simulink model "big2"  (R2023b)
settings: Solver=VariableStepAuto  StartTime=0.0  StopTime=500  RelTol=1e-3
libraries: simulink x2, aerolibasang x2, simulink_extras x2, aerolibanim x1
(part 2 of 3)

== matlab function big2/Subsystem1/Subsystem/MATLAB Function4 ==
  data: F input; V_dot output; g input; m input; theta input; psi input; P input; R input; U input; W input
function V_dot = fcn(F,g,m,theta,psi,P,R,U,W)
    if m == 0
        V_dot = NaN;
        warning('Mass (m) is zero, returning NaN.');
        return;
    end
    % Ensure theta and psi are valid
    if isnan(theta) || isnan(psi)
        V_dot = NaN;
        warning('Theta or Psi is NaN, returning NaN.');
        return;
    end
    V_dot = P*W - R*U + g*cos(theta)*sin(psi) + F/m;
    % V_dot = 0;

== matlab function big2/Subsystem1/Subsystem/MATLAB Function5 ==
  data: F input; W_dot output; g input; m input; theta input; psi input; P input; Q input; U input; V input
function W_dot = fcn(F,g,m,theta,psi,P,Q,U,V)
W_dot = Q*U - P*V + g*cos(theta)*cos(psi) + F/m;

== matlab function big2/Subsystem1/Subsystem/MATLAB Function6 ==
  data: phi input; euler_rates output; theta input; P input; Q input; R input
function euler_rates = fcn(phi, theta, P, Q, R)
if abs(cos(theta)) < 1e-6
    error('Theta is near ±pi/2, causing a singularity.');
end

T = [1, sin(phi)*tan(theta), cos(phi)*tan(theta);
     0, cos(phi), -sin(phi);
     0, sin(phi)/cos(theta), cos(phi)/cos(theta)];

angular_velocity = [P; Q; R];

euler_rates = T * angular_velocity;
end

== matlab function big2/Subsystem/Subsystem1/MATLAB Function ==
  data: alpha input; c_x output; el input
function c_x = compute_cx_fixed(alpha, el)
    data = [
    -0.099, -0.081, -0.081, -0.063, -0.025, 0.044, 0.097, 0.113, 0.145, 0.167, 0.174, 0.166;
    -0.048, -0.038, -0.040, -0.021, 0.016, 0.083, 0.127, 0.137, 0.162, 0.177, 0.179, 0.167;
    -0.022, -0.020, -0.021, -0.004, 0.032, 0.094, 0.128, 0.130, 0.154, 0.161, 0.155, 0.138;
    -0.040, -0.038, -0.039, -0.025, 0.006, 0.062, 0.087, 0.085, 0.100, 0.110, 0.104, 0.091;
    -0.083, -0.073, -0.076, -0.072, -0.046, 0.012, 0.024, 0.025, 0.043, 0.053, 0.047, 0.040
    ];
    % Scale Alpha and EL
    scaled_alpha = 0.2 * alpha;
    k = floor(scaled_alpha);
    k = max(-2, min(k, 8)); % Constrain within bounds
    da = scaled_alpha - k;
    l = k + sign(1.1 * da);
    l = max(-2, min(l, 8)); % Constrain within bounds

    % Adjust indices for 1-based indexing
    k_index = k + 3; % MATLAB 1-based (add 3 instead of 2 for [-2, 8])
    l_index = l + 3;

    % Scale EL
    scaled_el = el / 12.5;
    m = floor(scaled_el);
    m = max(-2, min(m, 2)); % Constrain within bounds
    de = scaled_el - m;
    n = m + sign(1.1 * de);
    n = max(-2, min(n, 2)); % Constrain within bounds

    % Adjust indices for 1-based indexing
    m_index = m + 3; % MATLAB 1-based (add 3 instead of 2 for [-2, 2])
    n_index = n + 3;

    % Ensure indices are within valid ranges
    assert(m_index >= 1 && m_index <= size(data, 1), 'm_index out of bounds');
    assert(n_index >= 1 && n_index <= size(data, 1), 'n_index out of bounds');
    assert(k_index >= 1 && k_index <= size(data, 2), 'k_index out of bounds');
    assert(l_index >= 1 && l_index <= size(data, 2), 'l_index out of bounds');

    % Interpolate values
    t = data(m_index, k_index); % Top-left
    u = data(n_index, k_index); % Bottom-left
    v = t + abs(da) * (data(m_index, l_index) - t); % Interpolation along top row
    w = u + abs(da) * (data(n_index, l_index) - u); % Interpolation along bottom row
    c_x = v + (w - v) * abs(de); % Final interpolation
end

== matlab function big2/Subsystem1/Subsystem/MATLAB Function7 ==
  data: U input; V input; W input; phi input; vel_dot output; theta input; psi input
function vel_dot = fcn(U, V, W, phi, theta, psi)
% This function computes [x_dot_e; y_dot_e; -h_dot] using the given equation.
% Inputs:
% U, V, W - Body frame velocities (m/s)
% phi     - Roll angle (rad)
% theta   - Pitch angle (rad)
% psi     - Yaw angle (rad)

% Rotation matrices
R_psi = [cos(psi), -sin(psi), 0;
         sin(psi),  cos(psi), 0;
         0,         0,        1];

R_theta = [cos(theta), 0, sin(theta);
           0,          1, 0;
          -sin(theta), 0, cos(theta)];

R_phi = [1, 0,       0;
         0, cos(phi), -sin(phi);
         0, sin(phi),  cos(phi)];

% Overall transformation matrix
R = R_psi * R_theta * R_phi;

% Body velocities vector
body_velocities = [U; V; W];

% Compute [x_dot_e; y_dot_e; -h_dot]
vel_dot = R * body_velocities;
end

== matlab function big2/Subsystem/Subsystem2/MATLAB Function ==
  data: alpha input; Cxq output
function Cxq = lookup_Cxq(alpha)
    % Initialize output
    Cxq = 0; % Ensure Cxq is scalar and fixed size

    % Declare persistent variables to hold constant data
    persistent alpha_values Cxq_values num_points

    if isempty(alpha_values)
        % Initialize the lookup table values as constants
        alpha_values = [-10, -5, 0, 5, 10, 15, 20, 25, 30, 35, 40, 45];
        Cxq_values  = [-0.267, -0.110, 0.308, 1.34, 2.08, 2.91, 2.76, 2.05, 1.50, 1.49, 1.83, 1.21];
        num_points = length(alpha_values);
    end

    % Handle values outside the table range
    if alpha <= alpha_values(1)
        Cxq = Cxq_values(1);
    elseif alpha >= alpha_values(num_points)
        Cxq = Cxq_values(num_points);
    else
        % Find the interval containing alpha
        idx = int32(1);
        for i = int32(1):(num_points - 1)
            if alpha_values(i) <= alpha && alpha < alpha_values(i+1)
                idx = i;
                break;
            end
        end

        % Get the two points for interpolation
        x1 = alpha_values(idx);
        x2 = alpha_values(idx + 1);
        y1 = Cxq_values(idx);
        y2 = Cxq_values(idx + 1);

        % Linear interpolation
        Cxq = y1 + ((y2 - y1) * (alpha - x1)) / (x2 - x1);
    end
end

== matlab function big2/Subsystem/Subsystem2/MATLAB Function1 ==
  data: alpha input; CYr output
function CYr = lookup_CYr(alpha)
    % Initialize output
    CYr = 0; % Ensure Cxq is scalar and fixed size

    % Declare persistent variables to hold constant data
    persistent alpha_values CYr_values num_points

    if isempty(alpha_values)
        % Initialize the lookup table values as constants
        alpha_values = [-Inf, -10, -5, 0, 5, 10, 15, 20, 25, 30, 35, 40, 45, Inf];
        CYr_values = [.882,.882, .852, .876, .958, .962, .974, .819, .483, .590, 1.21, -.493, -1.04, -1.04];
        num_points = length(alpha_values);
    end

    % Handle values outside the table range
    if alpha <= alpha_values(1)
        CYr = CYr_values(1);
    elseif alpha >= alpha_values(num_points)
        CYr = CYr_values(num_points);
    else
        % Find the interval containing alpha
        idx = int32(1);
        for i = int32(1):(num_points - 1)
            if alpha_values(i) <= alpha && alpha < alpha_values(i+1)
                idx = i;
                break;
            end
        end

        % Get the two points for interpolation
        x1 = alpha_values(idx);
        x2 = alpha_values(idx + 1);
        y1 = CYr_values(idx);
        y2 = CYr_values(idx + 1);

        % Linear interpolation
        CYr = y1 + ((y2 - y1) * (alpha - x1)) / (x2 - x1);
    end
end

== matlab function big2/Subsystem/Subsystem2/MATLAB Function2 ==
  data: alpha input; CYp output
function CYp = lookup_CYp(alpha)
    % Initialize output
    CYp = 0; % Ensure CYp is scalar and fixed size

    % Declare persistent variables to hold constant data
    persistent alpha_values CYp_values num_points

    if isempty(alpha_values)
        % Initialize the lookup table values as constants
        alpha_values = [-10, -5, 0, 5, 10, 15, 20, 25, 30, 35, 40, 45];
        CYp_values  = [-0.108, -0.188, 0.110, 0.258, 0.226, 0.344, 0.362, 0.611, 0.529, 0.298, -2.27, -2.27];
        num_points = length(alpha_values);
    end

    % Handle values outside the table range
    if alpha <= alpha_values(1)
        CYp = CYp_values(1);
    elseif alpha >= alpha_values(num_points)
        CYp = CYp_values(num_points);
    else
        % Find the interval containing alpha
        idx = int32(1);
        for i = int32(1):(num_points - 1)
            if alpha_values(i) <= alpha && alpha < alpha_values(i+1)
                idx = i;
                break;
            end
        end

        % Get the two points for interpolation
        x1 = alpha_values(idx);
        x2 = alpha_values(idx + 1);
        y1 = CYp_values(idx);
        y2 = CYp_values(idx + 1);

        % Linear interpolation
        CYp = y1 + ((y2 - y1) * (alpha - x1)) / (x2 - x1);
    end
end

== matlab function big2/Subsystem/Subsystem2/MATLAB Function3 ==
  data: alpha input; CZq output
function CZq = lookup_CZq(alpha)
    % Initialize output
    CZq = 0; % Ensure Cxq is scalar and fixed size

    % Declare persistent variables to hold constant data
    persistent alpha_values CZq_values num_points

    if isempty(alpha_values)
        % Initialize the lookup table values as constants
        alpha_values = [-Inf, -10, -5, 0, 5, 10, 15, 20, 25, 30, 35, 40, 45, Inf];
        CZq_values = [-8.80,-8.80, -25.8, -28.9, -31.4, -31.2, -30.7, -27.7, ...
                  -28.2, -29.0, -29.8, -38.3, -35.3, -35.3];
        num_points = length(alpha_values);
    end

    % Handle values outside the table range
    if alpha <= alpha_values(1)
        CZq = CZq_values(1);
    elseif alpha >= alpha_values(num_points)
        CZq = CZq_values(num_points);
    else
        % Find the interval containing alpha
        idx = int32(1);
        for i = int32(1):(num_points - 1)
            if alpha_values(i) <= alpha && alpha < alpha_values(i+1)
                idx = i;
                break;
            end
        end

        % Get the two points for interpolation
        x1 = alpha_values(idx);
        x2 = alpha_values(idx + 1);
        y1 = CZq_values(idx);
        y2 = CZq_values(idx + 1);

        % Linear interpolation
        CZq = y1 + ((y2 - y1) * (alpha - x1)) / (x2 - x1);
    end
end

== matlab function big2/Subsystem/Subsystem2/MATLAB Function4 ==
  data: alpha input; Clr output
function Clr = lookup_Clr(alpha)
    % Initialize output
    Clr = 0; % Ensure Cxq is scalar and fixed size

    % Declare persistent variables to hold constant data
    persistent alpha_values Clr_values num_points

    if isempty(alpha_values)
        % Initialize the lookup table values as constants
         alpha_values = [-Inf, -10, -5, 0, 5, 10, 15, 20, 25, 30, 35, 40, 45, Inf];
        Clr_values = [-0.126, -0.126, -0.026, 0.063, 0.113, 0.208, 0.230, 0.319, ...
                  0.437, 0.680, 0.100, 0.447, -0.330, -0.330];
        num_points = length(alpha_values);
    end

    % Handle values outside the table range
    if alpha <= alpha_values(1)
        Clr = Clr_values(1);
    elseif alpha >= alpha_values(num_points)
        Clr = Clr_values(num_points);
    else
        % Find the interval containing alpha
        idx = int32(1);
        for i = int32(1):(num_points - 1)
            if alpha_values(i) <= alpha && alpha < alpha_values(i+1)
                idx = i;
                break;
            end
        end

        % Get the two points for interpolation
        x1 = alpha_values(idx);
        x2 = alpha_values(idx + 1);
        y1 = Clr_values(idx);
        y2 = Clr_values(idx + 1);

        % Linear interpolation
        Clr = y1 + ((y2 - y1) * (alpha - x1)) / (x2 - x1);
    end
end

== matlab function big2/Subsystem/Subsystem2/MATLAB Function5 ==
  data: alpha input; Clp output
function Clp = lookup_Clp(alpha)
    % Initialize output
    Clp = 0; % Ensure Cxq is scalar and fixed size

    % Declare persistent variables to hold constant data
    persistent alpha_values Clp_values num_points

    if isempty(alpha_values)
        % Initialize the lookup table values as constants
         alpha_values = [-Inf, -10, -5, 0, 5, 10, 15, 20, 25, 30, 35, 40, 45, Inf];
        Clp_values = [-0.360, -0.360, -0.359, -0.443, -0.420, -0.383, -0.375, -0.329, ...
                  -0.294, -0.230, -0.210, -0.120, -0.100, -0.100];
        num_points = length(alpha_values);
    end

    % Handle values outside the table range
    if alpha <= alpha_values(1)
        Clp = Clp_values(1);
    elseif alpha >= alpha_values(num_points)
        Clp = Clp_values(num_points);
    else
        % Find the interval containing alpha
        idx = int32(1);
        for i = int32(1):(num_points - 1)
            if alpha_values(i) <= alpha && alpha < alpha_values(i+1)
                idx = i;
                break;
            end
        end

        % Get the two points for interpolation
        x1 = alpha_values(idx);
        x2 = alpha_values(idx + 1);
        y1 = Clp_values(idx);
        y2 = Clp_values(idx + 1);

        % Linear interpolation
        Clp = y1 + ((y2 - y1) * (alpha - x1)) / (x2 - x1);
    end
end

== matlab function big2/Subsystem/Subsystem2/MATLAB Function6 ==
  data: alpha input; Cmq output
function Cmq = lookup_Cmq(alpha)
    % Initialize output
    Cmq = 0; % Ensure Cxq is scalar and fixed size

    % Declare persistent variables to hold constant data
    persistent alpha_values Cmq_values num_points

    if isempty(alpha_values)
        % Initialize the lookup table values as constants
         alpha_values = [-Inf, -10, -5, 0, 5, 10, 15, 20, 25, 30, 35, 40, 45, Inf];
        Cmq_values = [-7.21, -7.21, -0.540, -5.23, -5.26, -6.11, -6.64, -5.69, ...
                  -6.00, -6.20, -6.40, -6.60, -6.00, -6.00];
    
        num_points = length(alpha_values);
    end

    % Handle values outside the table range
    if alpha <= alpha_values(1)
        Cmq = Cmq_values(1);
    elseif alpha >= alpha_values(num_points)
        Cmq = Cmq_values(num_points);
    else
        % Find the interval containing alpha
        idx = int32(1);
        for i = int32(1):(num_points - 1)
            if alpha_values(i) <= alpha && alpha < alpha_values(i+1)
                idx = i;
                break;
            end
        end

        % Get the two points for interpolation
        x1 = alpha_values(idx);
        x2 = alpha_values(idx + 1);
        y1 = Cmq_values(idx);
        y2 = Cmq_values(idx + 1);

        % Linear interpolation
        Cmq = y1 + ((y2 - y1) * (alpha - x1)) / (x2 - x1);
    end
end

== matlab function big2/Subsystem/Subsystem2/MATLAB Function7 ==
  data: alpha input; Cnr output
function Cnr = lookup_Cnr(alpha)
    % Initialize output
    Cnr = 0; % Ensure Cxq is scalar and fixed size

    % Declare persistent variables to hold constant data
    persistent alpha_values Cnr_values num_points

    if isempty(alpha_values)
        % Initialize the lookup table values as constants
         alpha_values = [-Inf, -10, -5, 0, 5, 10, 15, 20, 25, 30, 35, 40, 45, Inf];
        Cnr_values = [-0.380, -0.380, -0.363, -0.378, -0.386, -0.370, -0.453, -0.550, ...
                  -0.582, -0.595, -0.637, -1.02, -0.840, -0.840];
    
        num_points = length(alpha_values);
    end

    % Handle values outside the table range
    if alpha <= alpha_values(1)
        Cnr = Cnr_values(1);
    elseif alpha >= alpha_values(num_points)
        Cnr = Cnr_values(num_points);
    else
        % Find the interval containing alpha
        idx = int32(1);
        for i = int32(1):(num_points - 1)
            if alpha_values(i) <= alpha && alpha < alpha_values(i+1)
                idx = i;
                break;
            end
        end

        % Get the two points for interpolation
        x1 = alpha_values(idx);
        x2 = alpha_values(idx + 1);
        y1 = Cnr_values(idx);
        y2 = Cnr_values(idx + 1);

        % Linear interpolation
        Cnr = y1 + ((y2 - y1) * (alpha - x1)) / (x2 - x1);
    end
end

== matlab function big2/Subsystem/Subsystem2/MATLAB Function8 ==
  data: alpha input; Cnp output
function Cnp = lookup_Cnp(alpha)
    % Initialize output
    Cnp = 0; % Ensure Cxq is scalar and fixed size

    % Declare persistent variables to hold constant data
    persistent alpha_values Cnp_values num_points

    if isempty(alpha_values)
        % Initialize the lookup table values as constants
        alpha_values = [-Inf, -10, -5, 0, 5, 10, 15, 20, 25, 30, 35, 40, 45, Inf];
        Cnp_values = [0.061,0.061, 0.052, 0.052, -0.012, -0.013, -0.024, 0.050, ...
                  0.150, 0.130, 0.158, 0.240, 0.150, 0.150];
    
        num_points = length(alpha_values);
    end

    % Handle values outside the table range
    if alpha <= alpha_values(1)
        Cnp = Cnp_values(1);
    elseif alpha >= alpha_values(num_points)
        Cnp = Cnp_values(num_points);
    else
        % Find the interval containing alpha
        idx = int32(1);
        for i = int32(1):(num_points - 1)
            if alpha_values(i) <= alpha && alpha < alpha_values(i+1)
                idx = i;
                break;
            end
        end

        % Get the two points for interpolation
        x1 = alpha_values(idx);
        x2 = alpha_values(idx + 1);
        y1 = Cnp_values(idx);
        y2 = Cnp_values(idx + 1);

        % Linear interpolation
        Cnp = y1 + ((y2 - y1) * (alpha - x1)) / (x2 - x1);
    end
end

== matlab function big2/Subsystem/Subsystem1/MATLAB Function1 ==
  data: alpha input; c_z output; beta input; el input


function c_z = compute_cz(alpha, beta, el)
    data_CZ_updated_data_full = [
    0.770, 0.241, -0.100, -0.416, -0.731, -1.053, ...
    -1.366, -1.646, -1.917, -2.120, -2.248, -2.229
    ];
    
    % Map Alpha into indices and interpolate
    scaled_alpha = 0.2 * alpha;
    k = floor(scaled_alpha);
    k = max(-2, min(k, 8)); % Constrain within bounds
    da = scaled_alpha - k;
    l = k + sign(1.1 * da);
    l = max(-1, min(l, 8)); % Constrain within bounds

    % Adjust index for MATLAB (1-based indexing)
    k_index = k + 3;
    l_index = l + 3;

    % Calculate 's' using the provided formula
    s = data_CZ_updated_data_full(k_index) + abs(da) * ...
        (data_CZ_updated_data_full(l_index) - data_CZ_updated_data_full(k_index));
    c_z = s * (1 - (beta / 57.3)^2) - 0.19 * (el / 25.0);
end

== matlab function big2/Subsystem/Aero_moment_coef/MATLAB Function ==
  data: ail input; moment_coeffs output; rud input; B input; Vt input; force_coeffs input; euler_rates input; aero_moment_coeffs input; moment_stab_derivs input; ctrl_surf_coeffs input; cbar input; xcgr_xcg input
function moment_coeffs = compute_moment_coeffs(ail, rud, B, Vt, force_coeffs, euler_rates, aero_moment_coeffs, moment_stab_derivs, ctrl_surf_coeffs, cbar, xcgr_xcg)
    % Inputs:
    % ail                - Aileron deflection (degrees)
    % rud                - Rudder deflection (degrees)
    % B                  - Wing span (meters)
    % Vt                 - Total velocity (m/s)
    % force_coeffs       - Array [Cy_tot, Cz_tot]
    % euler_rates        - Array [P, Q, R] (roll, pitch, yaw rates)
    % aero_moment_coeffs - Array [Cl, Cm, Cn] (moment coefficients)
    % moment_stab_derivs - Array [Clr, Clp, Cmq, Cnr, Cnp] (stability derivatives)
    % ctrl_surf_coeffs   - Array [delta_Cl_a20, delta_Cl_r30, delta_Cn_a20, delta_Cn_r30]
    % cbar               - Mean aerodynamic chord (meters)
    % xcgr_xcg           - CG location relative to aerodynamic center
    
    moment_coeffs = zeros(1, 3); % Fixed size: 1x3 vector


    % Normalize control surface deflections
    norm_ail = ail / 21.5;
    norm_rud = rud / 30.0;
    B_over_2Vt = B / (2 * Vt);
    
    % Extract force coefficients
    Cy_tot = force_coeffs(2);
    Cz_tot = force_coeffs(3);
    
    % Extract Euler rates
    P = euler_rates(1);
    Q = euler_rates(2);
    R = euler_rates(3);
    
    % Extract aerodynamic moment coefficients
    Cl = aero_moment_coeffs(1);
    Cm = aero_moment_coeffs(2);
    Cn = aero_moment_coeffs(3);
    
    % Extract stability derivatives
    Clr = moment_stab_derivs(1);
    Clp = moment_stab_derivs(2);
    Cmq = moment_stab_derivs(3);
    Cnr = moment_stab_derivs(4);
    Cnp = moment_stab_derivs(5);
    
    % Extract control surface coefficients
    delta_Cl_a20 = ctrl_surf_coeffs(1);
    delta_Cl_r30 = ctrl_surf_coeffs(2);
    delta_Cn_a20 = ctrl_surf_coeffs(3);
    delta_Cn_r30 = ctrl_surf_coeffs(4);
    
    % Compute total coefficients
    Cl_tot = Cl ...
        + delta_Cl_a20 * norm_ail ...
        + delta_Cl_r30 * norm_rud ...
        + B_over_2Vt * Clp * P ...
        + B_over_2Vt * Clr * R;

    Cm_tot = Cm ...
        + (0.5 * cbar / Vt) * Cmq * Q ...
        + Cz_tot * xcgr_xcg;

    Cn_tot = Cn ...
        + delta_Cn_a20 * norm_ail ...
        + delta_Cn_r30 * norm_rud ...
        + B_over_2Vt * Cnp * P ...
        + B_over_2Vt * Cnr * R ...
        - (cbar / B) * Cy_tot * xcgr_xcg;
    
    % Output moment coefficients
    moment_coeffs = [Cl_tot, Cm_tot, Cn_tot];
end

== matlab function big2/Subsystem/MATLAB Function ==
  data: z input; T output; Vt input; qbar output; mach output
function [T, qbar, mach] = atmosphereModel(z, Vt)
    % atmosphereModel computes temperature, dynamic pressure, and Mach number
    % Inputs:
    %   z  - Altitude (meters)
    %   Vt - True airspeed (m/s)
    % Outputs:
    %   T     - Temperature (Kelvin)
    %   qbar  - Dynamic pressure (Pa)
    %   mach  - Mach number

    % Constants
    T0 = 288.15;         % Sea level standard temperature (Kelvin)
    rho0 = 1.225;        % Sea level standard density (kg/m^3)
    g0 = 9.80665;        % Gravitational acceleration (m/s^2)
    R = 287.05;          % Specific gas constant for air (J/(kg·K))
    gamma_air = 1.4;     % Ratio of specific heats for air

    % Compute temperature
    T = T0 - 0.0065 * min(max(z, 0), 11000);

    % Compute dynamic pressure (qbar)
    qbar = 0.5 * rho0 * Vt^2 * exp((z * g0) / (R * T));

    % Compute Mach number
    mach = Vt / sqrt(gamma_air * R * T);
end

== matlab function big2/Subsystem/Subsystem3/MATLAB Function1 ==
  data: alpha input; DLDA output; beta input
% function DLDA = ddo_lookup(alpha, beta)
%     % Initialize output
%     DLDA = 0; % Ensure DLDN is scalar and fixed size
% 
%     % Declare persistent variables to hold constant data
%     persistent alpha_values beta_values data num_alpha num_beta
% 
%     if isempty(alpha_values)
%         % Initialize alpha and beta values in the table
%         alpha_values = [-10, -5, 0, 5, 10, 15, 20, 25, 30, 35, 40, 45];
%         beta_values  = [-30, -20, -10, 0, 10, 20, 30];
% 
%         num_alpha = length(alpha_values);
%         num_beta = length(beta_values);
% 
%         % Data matrix corresponding to beta (rows) and alpha (columns)
%         data = [
%         -0.041, -0.052, -0.053, -0.056, -0.050, -0.056, -0.082, -0.059, -0.042, -0.038, -0.027, -0.017; % Row for beta = -30°
%         -0.041, -0.053, -0.053, -0.053, -0.050, -0.051, -0.066, -0.043, -0.038, -0.027, -0.023, -0.016; % Row for beta = -20°
%         -0.042, -0.053, -0.052, -0.051, -0.049, -0.049, -0.043, -0.035, -0.026, -0.016, -0.018, -0.014; % Row for beta = -10°
%         -0.040, -0.052, -0.051, -0.052, -0.048, -0.048, -0.042, -0.037, -0.031, -0.026, -0.017, -0.012; % Row for beta = 0°
%         -0.043, -0.049, -0.048, -0.049, -0.043, -0.042, -0.042, -0.036, -0.025, -0.021, -0.016, -0.011; % Row for beta = 10°
%         -0.044, -0.048, -0.048, -0.047, -0.042, -0.041, -0.020, -0.028, -0.013, -0.014, -0.011, -0.010; % Row for beta = 20°
%         -0.043, -0.049, -0.047, -0.045, -0.042, -0.037, -0.003, -0.013, -0.010, -0.003, -0.007, -0.008; % Row for beta = 30°
%     ];
%     end
% 
%     % Ensure alpha is within the range; if not, use the closest value
%     alpha_index = int32(1);
%     min_alpha_diff = abs(alpha - alpha_values(1));
%     for i = int32(2):int32(num_alpha)
%         current_diff = abs(alpha - alpha_values(i));
%         if current_diff < min_alpha_diff
%             min_alpha_diff = current_diff;
%             alpha_index = i;
%         end
%     end
% 
%     % Ensure beta is within the range; if not, use the closest value
%     beta_index = int32(1);
%     min_beta_diff = abs(beta - beta_values(1));
%     for i = int32(2):int32(num_beta)
%         current_diff = abs(beta - beta_values(i));
%         if current_diff < min_beta_diff
%             min_beta_diff = current_diff;
%             beta_index = i;
%         end
%     end
% 
%     % Retrieve the corresponding value from the data table
%     DLDA = data(beta_index, alpha_index);
% end

function DLDA = ddo_lookup(alpha, beta)
    % Initialize output
    DLDA = 0; % Ensure DLDA is scalar and fixed size

    % Declare persistent variables to hold constant data
    persistent alpha_values beta_values data num_alpha num_beta

    if isempty(alpha_values)
        % Initialize alpha and beta values in the table
        alpha_values = [-10, -5, 0, 5, 10, 15, 20, 25, 30, 35, 40, 45];
        beta_values  = [-30, -20, -10, 0, 10, 20, 30];

        num_alpha = length(alpha_values);
        num_beta = length(beta_values);

        % Data matrix corresponding to beta (rows) and alpha (columns)
        data = [
            -0.041, -0.052, -0.053, -0.056, -0.050, -0.056, -0.082, -0.059, -0.042, -0.038, -0.027, -0.017;
            -0.041, -0.053, -0.053, -0.053, -0.050, -0.051, -0.066, -0.043, -0.038, -0.027, -0.023, -0.016;
            -0.042, -0.053, -0.052, -0.051, -0.049, -0.049, -0.043, -0.035, -0.026, -0.016, -0.018, -0.014;
            -0.040, -0.052, -0.051, -0.052, -0.048, -0.048, -0.042, -0.037, -0.031, -0.026, -0.017, -0.012;
            -0.043, -0.049, -0.048, -0.049, -0.043, -0.042, -0.042, -0.036, -0.025, -0.021, -0.016, -0.011;
            -0.044, -0.048, -0.048, -0.047, -0.042, -0.041, -0.020, -0.028, -0.013, -0.014, -0.011, -0.010;
            -0.043, -0.049, -0.047, -0.045, -0.042, -0.037, -0.003, -0.013, -0.010, -0.003, -0.007, -0.008;
        ];
    end

    % Handle out-of-range alpha values
    if alpha <= alpha_values(1)
        alpha_lower = alpha_values(1);
        alpha_upper = alpha_values(1);
        alpha_idx_lower = int32(1);
        alpha_idx_upper = int32(1);
    elseif alpha >= alpha_values(num_alpha)
        alpha_lower = alpha_values(num_alpha);
        alpha_upper = alpha_values(num_alpha);
        alpha_idx_lower = int32(num_alpha);
        alpha_idx_upper = int32(num_alpha);
    else
        % Find indices for alpha
        alpha_idx_lower = int32(1);
        alpha_idx_upper = int32(1);
        for i = int32(1):(num_alpha - 1)
            if alpha_values(i) <= alpha && alpha < alpha_values(i+1)
                alpha_idx_lower = i;
                alpha_idx_upper = i + 1;
                break;
            end
        end
        alpha_lower = alpha_values(alpha_idx_lower);
        alpha_upper = alpha_values(alpha_idx_upper);
    end

    % Handle out-of-range beta values
    if beta <= beta_values(1)
        beta_lower = beta_values(1);
        beta_upper = beta_values(1);
        beta_idx_lower = int32(1);
        beta_idx_upper = int32(1);
    elseif beta >= beta_values(num_beta)
        beta_lower = beta_values(num_beta);
        beta_upper = beta_values(num_beta);
        beta_idx_lower = int32(num_beta);
        beta_idx_upper = int32(num_beta);
    else
        % Find indices for beta
        beta_idx_lower = int32(1);
        beta_idx_upper = int32(1);
        for i = int32(1):(num_beta - 1)
            if beta_values(i) <= beta && beta < beta_values(i+1)
                beta_idx_lower = i;
                beta_idx_upper = i + 1;
                break;
            end
        end
        beta_lower = beta_values(beta_idx_lower);
        beta_upper = beta_values(beta_idx_upper);
    end

    % Get the four surrounding data points for bilinear interpolation
    Q11 = data(beta_idx_lower, alpha_idx_lower);
    Q12 = data(beta_idx_lower, alpha_idx_upper);
    Q21 = data(beta_idx_upper, alpha_idx_lower);
    Q22 = data(beta_idx_upper, alpha_idx_upper);

    % Perform bilinear interpolation
    if (alpha_upper - alpha_lower) == 0 && (beta_upper - beta_lower) == 0
        % Point lies exactly on a data point
        DLDA = data(beta_idx_lower, alpha_idx_lower);
    elseif (alpha_upper - alpha_lower) == 0
        % Interpolate in beta direction only
        DLDA = Q11 + ((beta - beta_lower) / (beta_upper - beta_lower)) * (Q21 - Q11);
    elseif (beta_upper - beta_lower) == 0
        % Interpolate in alpha direction only
        DLDA = Q11 + ((alpha - alpha_lower) / (alpha_upper - alpha_lower)) * (Q12 - Q11);
    else
        % Full bilinear interpolation
        DLDA = (1 / ((alpha_upper - alpha_lower) * (beta_upper - beta_lower))) * ...
               (Q11 * (alpha_upper - alpha) * (beta_upper - beta) + ...
                Q21 * (alpha - alpha_lower) * (beta_upper - beta) + ...
                Q12 * (alpha_upper - alpha) * (beta - beta_lower) + ...
                Q22 * (alpha - alpha_lower) * (beta - beta_lower));
    end
end

== matlab function big2/Subsystem/Subsystem3/MATLAB Function2 ==
  data: alpha input; DLDN output; beta input
% function DLDN = lookup_DLDN(alpha, beta)
%     % Initialize output
%     DLDN = 0; % Ensure DLDN is scalar and fixed size
% 
%     % Declare persistent variables to hold constant data
%     persistent alpha_values beta_values data num_alpha num_beta
% 
%     if isempty(alpha_values)
%         % Initialize alpha and beta values in the table
%         alpha_values = [-10, -5, 0, 5, 10, 15, 20, 25, 30, 35, 40, 45];
%         beta_values  = [-30, -20, -10, 0, 10, 20, 30];
% 
%         num_alpha = length(alpha_values);
%         num_beta = length(beta_values);
% 
%         % Data matrix corresponding to beta (rows) and alpha (columns)
%         data = [
%             0.005,  0.017,  0.014,  0.010, -0.005,  0.009,  0.019,  0.005,  0.000, -0.005, -0.011,  0.008; % Beta = -30°
%             0.007,  0.016,  0.014,  0.014,  0.013,  0.009,  0.012,  0.005,  0.000,  0.004,  0.009,  0.007; % Beta = -20°
%             0.013,  0.013,  0.011,  0.012,  0.011,  0.009,  0.008,  0.005, -0.002,  0.005,  0.003,  0.005; % Beta = -10°
%             0.018,  0.015,  0.015,  0.014,  0.014,  0.014,  0.014,  0.015,  0.013,  0.011,  0.006,  0.001; % Beta = 0°
%             0.015,  0.014,  0.013,  0.013,  0.012,  0.011,  0.011,  0.010,  0.008,  0.008,  0.007,  0.003; % Beta = 10°
%             0.021,  0.011,  0.010,  0.011,  0.010,  0.009,  0.008,  0.010,  0.006,  0.005,  0.000,  0.001; % Beta = 20°
%             0.023,  0.010,  0.011,  0.011,  0.011,  0.010,  0.008,  0.010,  0.006,  0.014,  0.020,  0.000; % Beta = 30°
%         ];
%     end
% 
%     % Ensure alpha is within the range; if not, use the closest value
%     alpha_index = int32(1);
%     min_alpha_diff = abs(alpha - alpha_values(1));
%     for i = int32(2):int32(num_alpha)
%         current_diff = abs(alpha - alpha_values(i));
%         if current_diff < min_alpha_diff
%             min_alpha_diff = current_diff;
%             alpha_index = i;
%         end
%     end
% 
%     % Ensure beta is within the range; if not, use the closest value
%     beta_index = int32(1);
%     min_beta_diff = abs(beta - beta_values(1));
%     for i = int32(2):int32(num_beta)
%         current_diff = abs(beta - beta_values(i));
%         if current_diff < min_beta_diff
%             min_beta_diff = current_diff;
%             beta_index = i;
%         end
%     end
% 
%     % Retrieve the corresponding value from the data table
%     DLDN = data(beta_index, alpha_index);
% end

function DLDN = lookup_DLDN(alpha, beta)
    % Initialize output
    DLDN = 0; % Ensure DLDN is scalar and fixed size

    % Declare persistent variables to hold constant data
    persistent alpha_values beta_values data num_alpha num_beta

    if isempty(alpha_values)
        % Initialize alpha and beta values in the table
        alpha_values = [-10, -5, 0, 5, 10, 15, 20, 25, 30, 35, 40, 45];
        beta_values  = [-30, -20, -10, 0, 10, 20, 30];

        num_alpha = length(alpha_values);
        num_beta = length(beta_values);

        % Data matrix corresponding to beta (rows) and alpha (columns)
        data = [
            0.005,  0.017,  0.014,  0.010, -0.005,  0.009,  0.019,  0.005,  0.000, -0.005, -0.011,  0.008;
            0.007,  0.016,  0.014,  0.014,  0.013,  0.009,  0.012,  0.005,  0.000,  0.004,  0.009,  0.007;
            0.013,  0.013,  0.011,  0.012,  0.011,  0.009,  0.008,  0.005, -0.002,  0.005,  0.003,  0.005;
            0.018,  0.015,  0.015,  0.014,  0.014,  0.014,  0.014,  0.015,  0.013,  0.011,  0.006,  0.001;
            0.015,  0.014,  0.013,  0.013,  0.012,  0.011,  0.011,  0.010,  0.008,  0.008,  0.007,  0.003;
            0.021,  0.011,  0.010,  0.011,  0.010,  0.009,  0.008,  0.010,  0.006,  0.005,  0.000,  0.001;
            0.023,  0.010,  0.011,  0.011,  0.011,  0.010,  0.008,  0.010,  0.006,  0.014,  0.020,  0.000;
        ];
    end

    % Handle out-of-range alpha values
    if alpha <= alpha_values(1)
        alpha_lower = alpha_values(1);
        alpha_upper = alpha_values(1);
        alpha_idx_lower = int32(1);
        alpha_idx_upper = int32(1);
    elseif alpha >= alpha_values(num_alpha)
        alpha_lower = alpha_values(num_alpha);
        alpha_upper = alpha_values(num_alpha);
        alpha_idx_lower = int32(num_alpha);
        alpha_idx_upper = int32(num_alpha);
    else
        % Find indices for alpha
        alpha_idx_lower = int32(1);
        alpha_idx_upper = int32(1);
        for i = int32(1):(num_alpha - 1)
            if alpha_values(i) <= alpha && alpha < alpha_values(i+1)
                alpha_idx_lower = i;
                alpha_idx_upper = i + 1;
                break;
            end
        end
        alpha_lower = alpha_values(alpha_idx_lower);
        alpha_upper = alpha_values(alpha_idx_upper);
    end

    % Handle out-of-range beta values
    if beta <= beta_values(1)
        beta_lower = beta_values(1);
        beta_upper = beta_values(1);
        beta_idx_lower = int32(1);
        beta_idx_upper = int32(1);
    elseif beta >= beta_values(num_beta)
        beta_lower = beta_values(num_beta);
        beta_upper = beta_values(num_beta);
        beta_idx_lower = int32(num_beta);
        beta_idx_upper = int32(num_beta);
    else
        % Find indices for beta
        beta_idx_lower = int32(1);
        beta_idx_upper = int32(1);
        for i = int32(1):(num_beta - 1)
            if beta_values(i) <= beta && beta < beta_values(i+1)
                beta_idx_lower = i;
                beta_idx_upper = i + 1;
                break;
            end
        end
        beta_lower = beta_values(beta_idx_lower);
        beta_upper = beta_values(beta_idx_upper);
    end

    % Get the four surrounding data points for bilinear interpolation
    Q11 = data(beta_idx_lower, alpha_idx_lower);
    Q12 = data(beta_idx_lower, alpha_idx_upper);
    Q21 = data(beta_idx_upper, alpha_idx_lower);
    Q22 = data(beta_idx_upper, alpha_idx_upper);

    % Perform bilinear interpolation
    if (alpha_upper - alpha_lower) == 0 && (beta_upper - beta_lower) == 0
        % Point lies exactly on a data point
        DLDN = data(beta_idx_lower, alpha_idx_lower);
    elseif (alpha_upper - alpha_lower) == 0
        % Interpolate in beta direction only
        DLDN = Q11 + ((beta - beta_lower) / (beta_upper - beta_lower)) * (Q21 - Q11);
    elseif (beta_upper - beta_lower) == 0
        % Interpolate in alpha direction only
        DLDN = Q11 + ((alpha - alpha_lower) / (alpha_upper - alpha_lower)) * (Q12 - Q11);
    else
        % Full bilinear interpolation
        DLDN = (1 / ((alpha_upper - alpha_lower) * (beta_upper - beta_lower))) * ...
               (Q11 * (alpha_upper - alpha) * (beta_upper - beta) + ...
                Q21 * (alpha - alpha_lower) * (beta_upper - beta) + ...
                Q12 * (alpha_upper - alpha) * (beta - beta_lower) + ...
                Q22 * (alpha - alpha_lower) * (beta - beta_lower));
    end
end

== matlab function big2/Subsystem/Subsystem3/MATLAB Function3 ==
  data: alpha input; DNDA output; beta input
% function DNDA = ddo_lookup(alpha, beta)
%     % Initialize output
%     DNDA = 0; % Ensure DLDN is scalar and fixed size
% 
%     % Declare persistent variables to hold constant data
%     persistent alpha_values beta_values data num_alpha num_beta
% 
%     if isempty(alpha_values)
%         % Initialize alpha and beta values in the table
%         alpha_values = [-10, -5, 0, 5, 10, 15, 20, 25, 30, 35, 40, 45];
%         beta_values  = [-30, -20, -10, 0, 10, 20, 30];
% 
%         num_alpha = length(alpha_values);
%         num_beta = length(beta_values);
% 
%         % Data matrix corresponding to beta (rows) and alpha (columns)
%          data = [
%     0.001, -0.027, -0.017, -0.013, -0.012, -0.016,  0.001, ...
%     0.017,  0.011,  0.017,  0.008,  0.016; % Row for beta = -30°
% 
%     0.002, -0.014, -0.016, -0.016, -0.014, -0.019, -0.021, ...
%     0.002,  0.012,  0.015,  0.015,  0.011; % Row for beta = -20°
% 
%    -0.006, -0.008, -0.006, -0.006, -0.005, -0.008, -0.005, ...
%     0.007,  0.004,  0.007,  0.006,  0.006; % Row for beta = -10°
% 
%    -0.011, -0.011, -0.010, -0.009, -0.008, -0.006,  0.000, ...
%     0.004,  0.007,  0.010,  0.004,  0.010; % Row for beta = 0°
% 
%    -0.015, -0.015, -0.014, -0.012, -0.011, -0.008, -0.002, ...
%     0.002,  0.006,  0.012,  0.011,  0.011; % Row for beta = 10°
% 
%    -0.024, -0.010, -0.004, -0.002, -0.001,  0.003,  0.014, ...
%     0.006, -0.001,  0.004,  0.004,  0.006; % Row for beta = 20°
% 
%    -0.022,  0.002, -0.003, -0.005, -0.003, -0.001, -0.009, ...
%    -0.009, -0.001,  0.003, -0.002,  0.001; % Row for beta = 30°
% ];
%     end
% 
%     % Ensure alpha is within the range; if not, use the closest value
%     alpha_index = int32(1);
%     min_alpha_diff = abs(alpha - alpha_values(1));
%     for i = int32(2):int32(num_alpha)
%         current_diff = abs(alpha - alpha_values(i));
%         if current_diff < min_alpha_diff
%             min_alpha_diff = current_diff;
%             alpha_index = i;
%         end
%     end
% 
%     % Ensure beta is within the range; if not, use the closest value
%     beta_index = int32(1);
%     min_beta_diff = abs(beta - beta_values(1));
%     for i = int32(2):int32(num_beta)
%         current_diff = abs(beta - beta_values(i));
%         if current_diff < min_beta_diff
%             min_beta_diff = current_diff;
%             beta_index = i;
%         end
%     end
% 
%     % Retrieve the corresponding value from the data table
%     DNDA = data(beta_index, alpha_index);
% end

function DNDA = ddo_lookup(alpha, beta)
    % Initialize output
    DNDA = 0; % Ensure DNDA is scalar and fixed size

    % Declare persistent variables to hold constant data
    persistent alpha_values beta_values data num_alpha num_beta

    if isempty(alpha_values)
        % Initialize alpha and beta values in the table
        alpha_values = [-10, -5, 0, 5, 10, 15, 20, 25, 30, 35, 40, 45];
        beta_values  = [-30, -20, -10, 0, 10, 20, 30];

        num_alpha = length(alpha_values);
        num_beta = length(beta_values);

        % Data matrix corresponding to beta (rows) and alpha (columns)
        data = [
            0.001, -0.027, -0.017, -0.013, -0.012, -0.016,  0.001,  0.017,  0.011,  0.017,  0.008,  0.016; % Beta = -30°
            0.002, -0.014, -0.016, -0.016, -0.014, -0.019, -0.021,  0.002,  0.012,  0.015,  0.015,  0.011; % Beta = -20°
           -0.006, -0.008, -0.006, -0.006, -0.005, -0.008, -0.005,  0.007,  0.004,  0.007,  0.006,  0.006; % Beta = -10°
           -0.011, -0.011, -0.010, -0.009, -0.008, -0.006,  0.000,  0.004,  0.007,  0.010,  0.004,  0.010; % Beta = 0°
           -0.015, -0.015, -0.014, -0.012, -0.011, -0.008, -0.002,  0.002,  0.006,  0.012,  0.011,  0.011; % Beta = 10°
           -0.024, -0.010, -0.004, -0.002, -0.001,  0.003,  0.014,  0.006, -0.001,  0.004,  0.004,  0.006; % Beta = 20°
           -0.022,  0.002, -0.003, -0.005, -0.003, -0.001, -0.009, -0.009, -0.001,  0.003, -0.002,  0.001; % Beta = 30°
        ];
    end

    % Handle out-of-range alpha values
    if alpha <= alpha_values(1)
        alpha_lower = alpha_values(1);
        alpha_upper = alpha_values(1);
        alpha_idx_lower = int32(1);
        alpha_idx_upper = int32(1);
    elseif alpha >= alpha_values(num_alpha)
        alpha_lower = alpha_values(num_alpha);
        alpha_upper = alpha_values(num_alpha);
        alpha_idx_lower = int32(num_alpha);
        alpha_idx_upper = int32(num_alpha);
    else
        % Find indices for alpha
        alpha_idx_lower = int32(1);
        alpha_idx_upper = int32(1);
        for i = int32(1):(num_alpha - 1)
            if alpha_values(i) <= alpha && alpha < alpha_values(i+1)
                alpha_idx_lower = i;
                alpha_idx_upper = i + 1;
                break;
            end
        end
        alpha_lower = alpha_values(alpha_idx_lower);
        alpha_upper = alpha_values(alpha_idx_upper);
    end

    % Handle out-of-range beta values
    if beta <= beta_values(1)
        beta_lower = beta_values(1);
        beta_upper = beta_values(1);
        beta_idx_lower = int32(1);
        beta_idx_upper = int32(1);
    elseif beta >= beta_values(num_beta)
        beta_lower = beta_values(num_beta);
        beta_upper = beta_values(num_beta);
        beta_idx_lower = int32(num_beta);
        beta_idx_upper = int32(num_beta);
    else
        % Find indices for beta
        beta_idx_lower = int32(1);
        beta_idx_upper = int32(1);
        for i = int32(1):(num_beta - 1)
            if beta_values(i) <= beta && beta < beta_values(i+1)
                beta_idx_lower = i;
                beta_idx_upper = i + 1;
                break;
            end
        end
        beta_lower = beta_values(beta_idx_lower);
        beta_upper = beta_values(beta_idx_upper);
    end

    % Get the four surrounding data points for bilinear interpolation
    Q11 = data(beta_idx_lower, alpha_idx_lower);
    Q12 = data(beta_idx_lower, alpha_idx_upper);
    Q21 = data(beta_idx_upper, alpha_idx_lower);
    Q22 = data(beta_idx_upper, alpha_idx_upper);

    % Perform bilinear interpolation
    if (alpha_upper - alpha_lower) == 0 && (beta_upper - beta_lower) == 0
        % Point lies exactly on a data point
        DNDA = data(beta_idx_lower, alpha_idx_lower);
    elseif (alpha_upper - alpha_lower) == 0
        % Interpolate in beta direction only
        DNDA = Q11 + ((beta - beta_lower) / (beta_upper - beta_lower)) * (Q21 - Q11);
    elseif (beta_upper - beta_lower) == 0
        % Interpolate in alpha direction only
        DNDA = Q11 + ((alpha - alpha_lower) / (alpha_upper - alpha_lower)) * (Q12 - Q11);
    else
        % Full bilinear interpolation
        DNDA = (1 / ((alpha_upper - alpha_lower) * (beta_upper - beta_lower))) * ...
               (Q11 * (alpha_upper - alpha) * (beta_upper - beta) + ...
                Q21 * (alpha - alpha_lower) * (beta_upper - beta) + ...
                Q12 * (alpha_upper - alpha) * (beta - beta_lower) + ...
                Q22 * (alpha - alpha_lower) * (beta - beta_lower));
    end
end
